simulink model "mbed_arch_max_datalogger"  (R2015a)
settings: Solver=FixedStepDiscrete  SolverMode=SingleTasking  StartTime=0.0  StopTime=10.0  FixedStep=1e-3  RelTol=1e-3
libraries: mbed_targets_stm_arch_max x1
settings Model: Creator=oh  LastModifiedBy=oh
settings OptimizationCC: OptimizeModelRefInitCode=on  LifeSpan=1
settings HardwareCC: ProdLargestAtomicInteger=Long  ProdLargestAtomicFloat=Double  ProdEndianess=LittleEndian  ProdHWDeviceType=ARM Compatible->ARM Cortex
settings RTWCC: SystemTargetFile=mbed.tlc  GenCodeOnly=on  TemplateMakefile=mbed.tmf  Description=Mbed Target (Embedded Target)  TargetLang=C++
settings CodeAppCC: IgnoreCustomStorageClasses=off
settings STFCustomTargetCC: CombineOutputUpdateFcns=on  SupportContinuousTime=off  SupportVariableSizeSignals=off  SystemTargetFile=mbed.tlc
settings ERTTargetCC: SupportContinuousTime=off  SupportVariableSizeSignals=off  ERTCustomFileTemplate=mbed_file_process.tlc

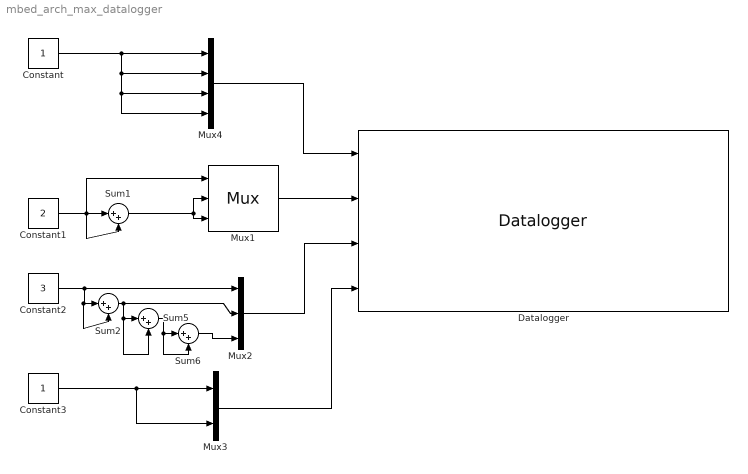
== system mbed_arch_max_datalogger ==
  Constant : Constant  OutDataTypeStr=uint8
  Constant1 : Constant  Value=2  OutDataTypeStr=int16
  Constant2 : Constant  Value=3
  Constant3 : Constant  OutDataTypeStr=boolean
  Datalogger : mbed_targets_stm_arch_max/Datalogger  TypeInputPorts={'uint8' 4 'int16' 3 'double' 3 'bool' 2}  SampleTime=-1  errEn=off  mosi_port=C  mosi_pin=3  miso_port=C  miso_pin=2  sclk_port=B  sclk_pin=10  cs_port=E  cs_pin=2
  Mux1 : Mux  Inputs=3
      settings: DisplayOption=signals
  Mux2 : Mux  Inputs=3
  Mux3 : Mux  Inputs=2
  Mux4 : Mux
  Sum{1..2,5..6} (4 alike) : Sum  Inputs=|++
  wires:
  Sum1/1 -> Mux1/2, Mux1/3
  Sum2/1 -> Mux2/2, Sum5/2, Sum5/1
  Constant1/1 -> Sum1/2, Sum1/1, Mux1/1
  Constant2/1 -> Mux2/1, Sum2/2, Sum2/1
  Sum5/1 -> Sum6/2, Sum6/1
  Constant3/1 -> Mux3/2, Mux3/1
  Sum6/1 -> Mux2/3
  Mux2/1 -> Datalogger/3
  Mux1/1 -> Datalogger/2
  Mux3/1 -> Datalogger/4
  Constant/1 -> Mux4/4, Mux4/3, Mux4/2, Mux4/1
  Mux4/1 -> Datalogger/1
